simulink model "rest_spike_bistability"  (R2015b)
settings: Solver=ode45  StartTime=0.0  StopTime=10000  RelTol=1e-3
values from neighbouring files (symbols this model uses):
  alpha = 0.25    [three_time_scale.m]
  alpha_delay1 = 4000    [three_time_scale.m]
  alpha_delay2 = 7000    [three_time_scale.m]
  alpha_max = 1    [three_time_scale.m]
  alpha_period = t_max    (= 10000)    [three_time_scale.m]
  alpha_width = 1    [three_time_scale.m]
  delta = 0.5    [three_time_scale.m]
  fast_plant_X0 = -1    [three_time_scale.m]
  gamma = 1    [three_time_scale.m]
  slow_plant_X0 = -2    [three_time_scale.m]
  ts = 1    [three_time_scale.m]
undefined symbols (not defined in the file or in its folder): beta2
settings Model: Creator=rajiv  LastModifiedBy=rajiv
settings HardwareCC: ProdWordSize=32  ProdHWDeviceType=Specified

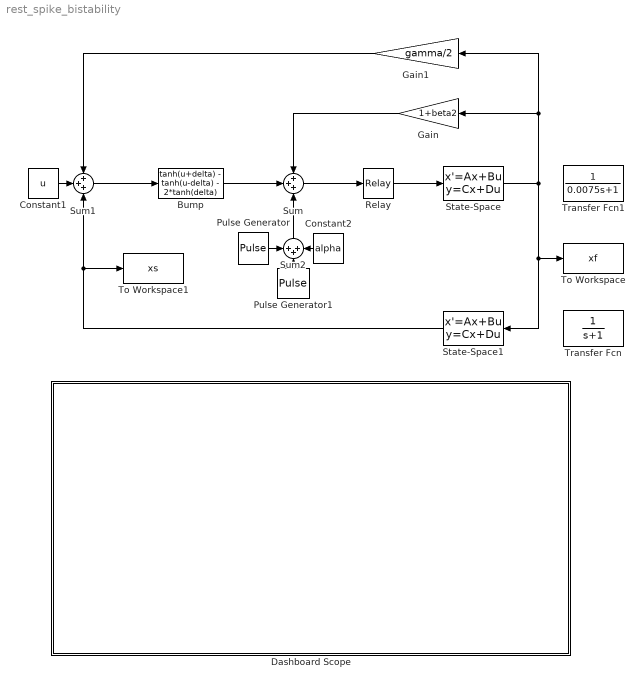
== system rest_spike_bistability ==
  Bump : Fcn  Expr="tanh(u+delta) -  tanh(u-delta) - 2*tanh(delta)"
  Constant1 : Constant  Value=u
  Constant2 : Constant  Value=alpha
  Dashboard Scope : Subsystem  DialogController=hmiCreateDDGDialog  IsWebBlock=on  mask(MWDashboardBlock){webBlockId=68aa9a0c-b9c9-4419-83a5-8653b2e17286, webBlockType=sdiscope, ShowInitialText=on, HMISrcModelName=rest_spike_bistability}
      mask prompts: webBlockId "WebBlock Id"; webBlockType "WebBlock Type"; HMISrcModelName "Source Model"
      mask Help: helpview([docroot '/mapfiles/simulink.map'], 'hmi_scope')
      mask Display:
      | if strcmp(get_param(bdroot(gcb),'BlockDiagramType'), 'library')
      |     image([(matlabroot) '/toolbox/simulink/hmi/icons/DashboardScope.png']);
      | end
  Gain : Gain  Gain=1+beta2
  Gain1 : Gain  Gain=gamma/2
  Pulse Generator : DiscretePulseGenerator  PulseType=Time based  Amplitude=alpha_max  Period=alpha_period  PulseWidth=alpha_width  PhaseDelay=alpha_delay1
  Pulse Generator1 : DiscretePulseGenerator  PulseType=Time based  Amplitude=-1*alpha_max  Period=alpha_period  PulseWidth=alpha_width  PhaseDelay=alpha_delay2
  Relay : Relay  OnSwitchValue=0  OffSwitchValue=0  OffOutputValue=-1
  State-Space : StateSpace  A=-1/tf  B=1/tf  D=0  X0=fast_plant_X0
  State-Space1 : StateSpace  A=-1/ts  B=1/ts  D=0  X0=slow_plant_X0
  Sum : Sum  Inputs=+++
  Sum1 : Sum  Inputs=+++
  Sum2 : Sum  Inputs=+++
  To Workspace : ToWorkspace  VariableName=xf  SaveFormat=Timeseries  SampleTime=-1
  To Workspace1 : ToWorkspace  VariableName=xs  SaveFormat=Timeseries  SampleTime=-1
  Transfer Fcn : TransferFcn  Denominator=[1 1]
  Transfer Fcn1 : TransferFcn  Denominator=[0.0075 1]
  wires:
  Sum/1 -> Relay/1
  Gain/1 -> Sum/1
  State-Space1/1 -> To Workspace1/1, Sum1/3
  Gain1/1 -> Sum1/1
  Constant1/1 -> Sum1/2
  Relay/1 -> State-Space/1
  State-Space/1 -> To Workspace/1, State-Space1/1, Gain/1, Gain1/1
  Constant2/1 -> Sum2/3
  Pulse Generator/1 -> Sum2/1
  Sum2/1 -> Sum/3
  Pulse Generator1/1 -> Sum2/2
  Bump/1 -> Sum/2
  Sum1/1 -> Bump/1

== system rest_spike_bistability/Dashboard Scope ==
